simulink model "washing_machine"  (R2024b)
settings: Solver=VariableStepAuto  StartTime=0.0  StopTime=50  RelTol=1e-3
settings Model: Creator=shrey  LastModifiedBy=shrey

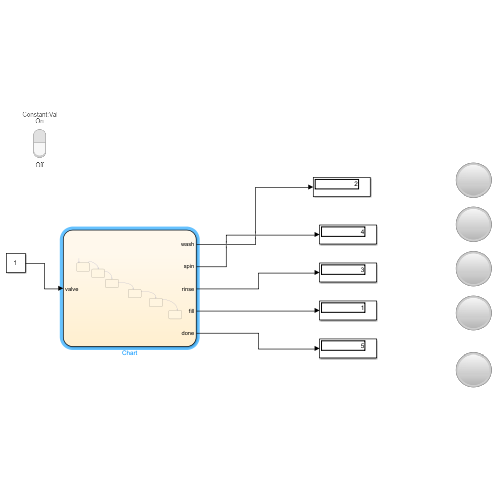
[thumbnail: Simulink's stored preview of the top-level diagram]
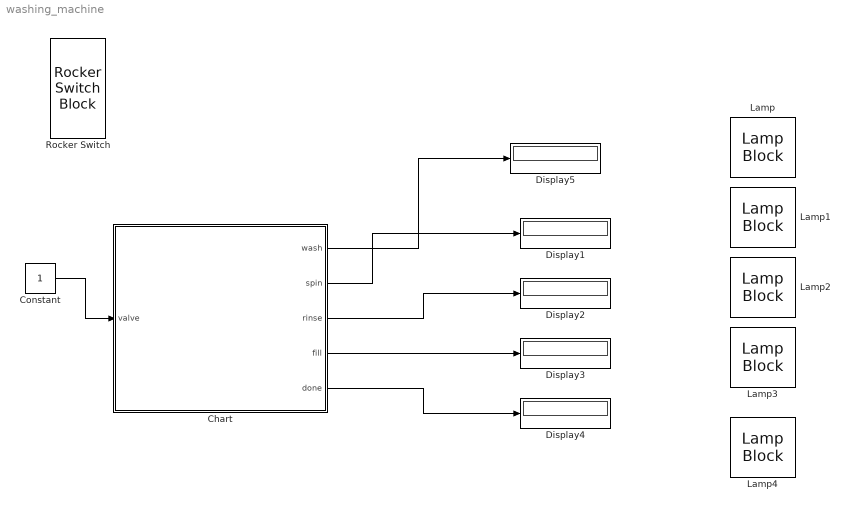
== system washing_machine ==
  Chart : Stateflow chart  TreatAsAtomicUnit=on
  Constant : Constant
  Display{1..5} (5 alike) : Display
  Lamp{,1..4} (5 alike) : LampBlock  LabelPosition=Hide
  Rocker Switch : RockerSwitchBlock
      settings: Values={{'Off', 'On'}, [0 1]}
  wires:
  Constant/1 -> Chart/1(valve)
  Chart/1(wash) -> Display5/1
  Chart/2(spin) -> Display1/1
  Chart/3(rinse) -> Display2/1
  Chart/4(fill) -> Display3/1
  Chart/5(done) -> Display4/1

== stateflow chart washing_machine/Chart ==
  state valve
  state fill
    entry:
    fill=1
  state wash
    entry:
    wash=2
  state rinse
    entry:
    rinse=3
  state spin
    entry:
    spin=4
  state done
    entry:
    done=5
  (default) -> valve
  valve -> fill : [valve==1]
  fill -> wash : [after(10,sec)]
  wash -> rinse : [after(10,sec)]
  rinse -> spin : [after(10,sec)]
  spin -> done : [after(10,sec)]
  data: wash output; spin output; rinse output; fill output; done output; valve input
